simulink library "allblocks_alteradspbuilder2"  (Simulink 7.6)
settings: Solver=ode45  StartTime=0.0  StopTime=10.0  RelTol=1e-3
InitFcn:
  | %% DSPBuilder Start
  | alt_dspbuilder_update_model(bdroot)
  | %% DSPBuilder End
undefined symbols (not defined in the file): alt_dspbuilder_internal_AvalonSTPFC_generate, alt_dspbuilder_internal_init_altlab_flow, alt_dspbuilder_internal_init_blackbox_flow, alt_dspbuilder_internal_initfcn_base_clock, alt_dspbuilder_internal_initfcn_clock, alt_dspbuilder_internal_initfcn_pll, alt_dspbuilder_load_block, alt_dspbuilder_update_external_RAM, Inferred
libraries: allblocks_alteradspbuilder2 x15
(part 4 of 4)

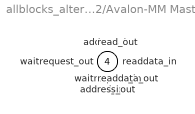
== system allblocks_alteradspbuilder2/Avalon-MM Master ==
  waitrequest_in : Inport
  address_in : Inport  Port=2
  read_in : Inport  Port=3
  readdata_in : Inport  Port=4
  waitrequest_out : Outport
  address_out : Outport  Port=2
  read_out : Outport  Port=3
  readdata_out : Outport  Port=4
  wires:
  ? -> ?

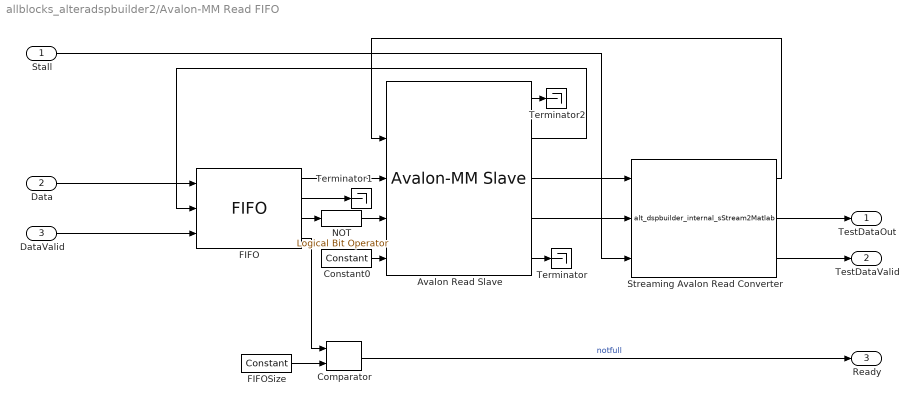
== system allblocks_alteradspbuilder2/Avalon-MM Read FIFO ==
  Stall : Inport
  Data : Inport  Port=2
  DataValid : Inport  Port=3
  Avalon Read Slave : allblocks_alteradspbuilder2/Avalon-MM Slave  SystemSampleTime=-1  iofile=D:\allblocks%5Falteradspbuilder2_Avalon-MM+Read+FIFO_Avalon+Read+Slave_address.salt,D:\allblocks%5Falteradspbuilder2_Avalon-MM+Read+FIFO_Avalon+Read+Slave_read.salt,D:\allblocks%5Falteradspbuilder2_Avalon-MM+Read+FIFO_Avalon+Read+Slave_readdata.capture,D:\allblocks%5Falteradspbuilder2_Avalon-MM+Read+FIFO_Avalon+Read+Slave_dataavailable.capture,D:\allblocks%5Falteradspbuilder2_Avalon-MM+Read+FIFO_Avalon+Read+Slave_endofpacket.capture,  SpecifyClock=off  clock=clock  addrWidth=2  addrAlignment=Dynamic  addrType=Read  BusType=Signed Integer  bwl=bwl  bwr=bwr  byteEnable=off  flowCtrl=on  pipeline=off  waitStateFormat=Fixed  readWaitStateCycles=0  writeWaitStateCycles=0  readLatencyFormat=Fixed  readLatencyCycles=0  burst=off  maxBurst=burst  irq=off  receiveBeginTransfer=off  useChipSelect=off  externalType=Inferred  PORTTYPE=Output
  Comparator : allblocks_alteradspbuilder2/Comparator  direction=a < b
  Constant0 : allblocks_alteradspbuilder2/Constant  mask_cst=0  BusType=Single Bit  bwl=1  bwr=0  SpecifyClock=off
  FIFO : allblocks_alteradspbuilder2/FIFO  numwords=depth  BusType=Signed Integer  bwl=bwl  bwr=bwr  ram_type=AUTO  use_sclr=off  use_les_only=off  showahead_mode=off
  FIFOSize : allblocks_alteradspbuilder2/Constant  mask_cst=depth - 2  BusType=Unsigned Integer  bwl=ceil(log2(depth -1))  bwr=0  SpecifyClock=off
  NOT : allblocks_alteradspbuilder2/Logical Bit Operator  LogicalOperator=NOT  user_inputs=2
  Streaming Avalon Read Converter : S-Function  FunctionName=alt_dspbuilder_internal_sStream2Matlab  Parameters=-1  EnableBusSupport=off
      mask Display:
      | port_label('input', 1, 'ReadData');
      | port_label('input', 2, 'DataAvailable');
      | port_label('input', 3, 'Stall');
      | port_label('output', 1, 'Read');
      | port_label('output', 2, 'TestData');
      | port_label('output', 3, 'TestDataValid');
  Terminator : Terminator
  Terminator1 : Terminator
  Terminator2 : Terminator
  TestDataOut : Outport
  TestDataValid : Outport  Port=2
  Ready : Outport  Port=3
  wires:
  Avalon Read Slave/1 -> Terminator2/1
  FIFO/2 -> Terminator1/1
  FIFOSize/1 -> Comparator/2
  Avalon Read Slave/5 -> Terminator/1
  Avalon Read Slave/4 -> Streaming Avalon Read Converter/2
  Stall/1 -> Streaming Avalon Read Converter/3
  Comparator/1 -> Ready/1  "notfull"
  FIFO/4 -> Comparator/1
  Constant0/1 -> Avalon Read Slave/5
  Avalon Read Slave/3 -> Streaming Avalon Read Converter/1
  Streaming Avalon Read Converter/1 -> Avalon Read Slave/2
  Streaming Avalon Read Converter/3 -> TestDataValid/1
  Streaming Avalon Read Converter/2 -> TestDataOut/1
  Avalon Read Slave/2 -> FIFO/2
  FIFO/1 -> Avalon Read Slave/3
  Data/1 -> FIFO/1
  NOT/1 -> Avalon Read Slave/4
  FIFO/3 -> NOT/1
  DataValid/1 -> FIFO/3

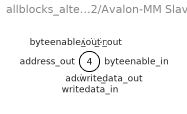
== system allblocks_alteradspbuilder2/Avalon-MM Slave ==
  address_in : Inport
  write_in : Inport  Port=2
  writedata_in : Inport  Port=3
  byteenable_in : Inport  Port=4
  address_out : Outport
  write_out : Outport  Port=2
  writedata_out : Outport  Port=3
  byteenable_out : Outport  Port=4
  wires:
  ? -> ?

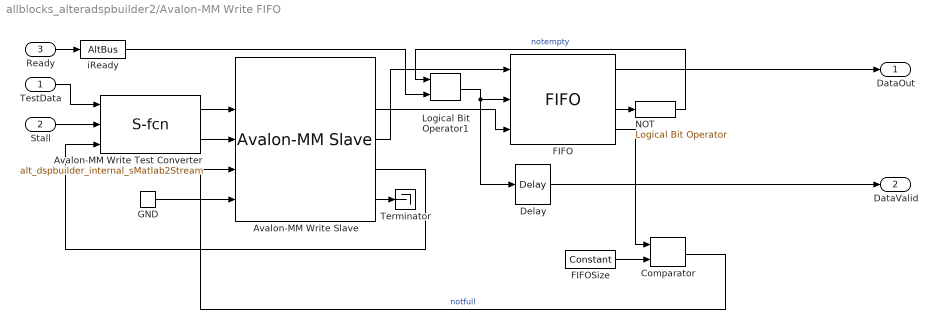
== system allblocks_alteradspbuilder2/Avalon-MM Write FIFO ==
  TestData : Inport
  Stall : Inport  Port=2
  Ready : Inport  Port=3
  Avalon-MM Write Slave : allblocks_alteradspbuilder2/Avalon-MM Slave  SystemSampleTime=-1  iofile=D:\allblocks%5Falteradspbuilder2_Avalon-MM+Write+FIFO_Avalon-MM+Write+Slave_address.salt,D:\allblocks%5Falteradspbuilder2_Avalon-MM+Write+FIFO_Avalon-MM+Write+Slave_write.salt,D:\allblocks%5Falteradspbuilder2_Avalon-MM+Write+FIFO_Avalon-MM+Write+Slave_writedata.salt,D:\allblocks%5Falteradspbuilder2_Avalon-MM+Write+FIFO_Avalon-MM+Write+Slave_readyfordata.capture,D:\allblocks%5Falteradspbuilder2_Avalon-MM+Write+FIFO_Avalon-MM+Write+Slave_endofpacket.capture,  SpecifyClock=off  clock=clock  addrWidth=2  addrAlignment=Dynamic  addrType=Write  BusType=Unsigned Integer  bwl=bwl  bwr=bwr  byteEnable=off  flowCtrl=on  pipeline=off  waitStateFormat=Fixed  readWaitStateCycles=0  writeWaitStateCycles=0  readLatencyFormat=Fixed  readLatencyCycles=0  burst=off  maxBurst=burst  irq=off  receiveBeginTransfer=off  useChipSelect=off  externalType=Inferred  PORTTYPE=Output
  Avalon-MM Write Test Converter : S-Function  FunctionName=alt_dspbuilder_internal_sMatlab2Stream  Parameters=-1 1000000  EnableBusSupport=off
      mask Display:
      | port_label('input', 1, 'TestData');
      | port_label('input', 2, 'Stall');
      | port_label('input', 3, 'Ready');
      | port_label('output', 1, 'Write');
      | port_label('output', 2, 'WriteData');
  Comparator : allblocks_alteradspbuilder2/Comparator  direction=a < b
  Delay : allblocks_alteradspbuilder2/Delay  pipeline=1  ClockPhase=1  use_ena=off  use_sclr=off
  FIFO : allblocks_alteradspbuilder2/FIFO  numwords=depth  BusType=Unsigned Integer  bwl=bwl  bwr=bwr  ram_type=AUTO  use_sclr=off  use_les_only=off  showahead_mode=off
  FIFOSize : allblocks_alteradspbuilder2/Constant  mask_cst=depth -2  BusType=Unsigned Integer  bwl=ceil(log2(depth-1))  bwr=0  SpecifyClock=off
  GND : allblocks_alteradspbuilder2/GND  SpecifyClock=off
  Logical Bit Operator1 : allblocks_alteradspbuilder2/Logical Bit Operator  LogicalOperator=AND  user_inputs=2
  NOT : allblocks_alteradspbuilder2/Logical Bit Operator  LogicalOperator=NOT  user_inputs=2
  Terminator : Terminator
  iReady : allblocks_alteradspbuilder2/AltBus  BusType=Single Bit  bwl=1  bwr=0  saturate=off  floatingPointInput=on  floatingPointOutput=on  logOutputs=off  logFile=D:\allblocks%5Falteradspbuilder2_Avalon-MM+Write+FIFO_iReady.fixedpointlog
  DataOut : Outport
  DataValid : Outport  Port=2
  wires:
  Logical Bit Operator1/1 -> Delay/1, FIFO/2
  FIFO/4 -> Comparator/1
  FIFOSize/1 -> Comparator/2
  Comparator/1 -> Avalon-MM Write Slave/4  "notfull"
  Avalon-MM Write Slave/5 -> Terminator/1
  Stall/1 -> Avalon-MM Write Test Converter/2
  Avalon-MM Write Test Converter/2 -> Avalon-MM Write Slave/3
  Delay/1 -> DataValid/1
  iReady/1 -> Logical Bit Operator1/2
  NOT/1 -> Logical Bit Operator1/1  "notempty"
  GND/1 -> Avalon-MM Write Slave/5
  TestData/1 -> Avalon-MM Write Test Converter/1
  Avalon-MM Write Slave/4 -> Avalon-MM Write Test Converter/3
  Avalon-MM Write Test Converter/1 -> Avalon-MM Write Slave/2
  FIFO/1 -> DataOut/1
  FIFO/3 -> NOT/1
  Avalon-MM Write Slave/2 -> FIFO/3
  Avalon-MM Write Slave/3 -> FIFO/1
  Ready/1 -> iReady/1

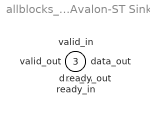
== system allblocks_alteradspbuilder2/Avalon-ST Sink ==
  data_in : Inport
  valid_in : Inport  Port=2
  ready_in : Inport  Port=3
  data_out : Outport
  valid_out : Outport  Port=2
  ready_out : Outport  Port=3
  wires:
  ? -> ?

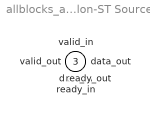
== system allblocks_alteradspbuilder2/Avalon-ST Source ==
  data_in : Inport
  valid_in : Inport  Port=2
  ready_in : Inport  Port=3
  data_out : Outport
  valid_out : Outport  Port=2
  ready_out : Outport  Port=3
  wires:
  ? -> ?
